simulink model "partH"  (R2018b)
settings: Solver=VariableStepAuto  StartTime=0.0  StopTime=10.0  RelTol=1e-3
settings Model: Creator=amir  LastModifiedBy=amir

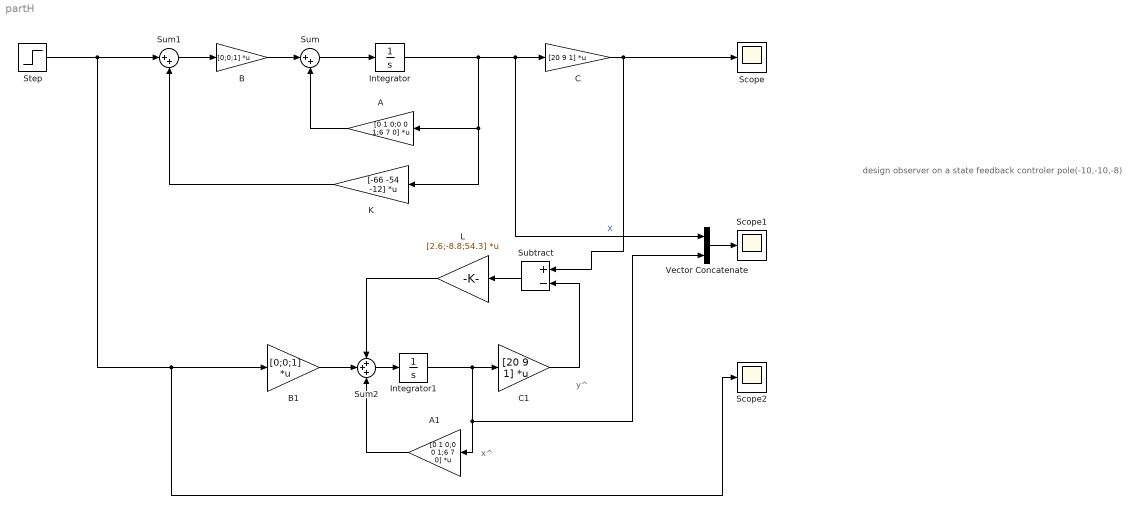
== system partH ==
  note: design observer on a
      | state feedback controler
      | pole(-10,-10,-8)
  note: x^
  note: y^
  A : Gain  Gain=[0 1 0;0 0 1;6 7 0]  Multiplication=Matrix(K*u) (u vector)
  A1 : Gain  Gain=[0 1 0;0 0 1;6 7 0]  Multiplication=Matrix(K*u) (u vector)
  B : Gain  Gain=[0;0;1]  Multiplication=Matrix(K*u) (u vector)
  B1 : Gain  Gain=[0;0;1]  Multiplication=Matrix(K*u) (u vector)
  C : Gain  Gain=[20 9 1]  Multiplication=Matrix(K*u) (u vector)
  C1 : Gain  Gain=[20 9 1]  Multiplication=Matrix(K*u) (u vector)
  Integrator : Integrator  InitialCondition=[1;1;1]
  Integrator1 : Integrator  InitialCondition=[1;1;1]
  K : Gain  Gain=[-66 -54 -12]  Multiplication=Matrix(K*u) (u vector)
  L : Gain  Gain=[2.6;-8.8;54.3]  Multiplication=Matrix(K*u) (u vector)
  Scope : Scope
  Scope1 : Scope
  Scope2 : Scope
  Step : Step  SampleTime=0
  Subtract : Sum  Inputs=+-
  Sum : Sum  Inputs=|++
  Sum1 : Sum  Inputs=|++
  Sum2 : Sum  Inputs=+++
  Vector Concatenate : Concatenate
  wires:
  Step/1 -> Scope2/1, B1/1, Sum1/1
  K/1 -> Sum1/2
  Sum1/1 -> B/1
  Integrator/1 -> Vector Concatenate/1, C/1, K/1, A/1  "X"
  Sum/1 -> Integrator/1
  C/1 -> Scope/1, Subtract/1
  A/1 -> Sum/2
  B/1 -> Sum/1
  B1/1 -> Sum2/2
  Sum2/1 -> Integrator1/1
  Vector Concatenate/1 -> Scope1/1
  A1/1 -> Sum2/3
  Integrator1/1 -> C1/1, Vector Concatenate/2, A1/1
  C1/1 -> Subtract/2
  Subtract/1 -> L/1
  L/1 -> Sum2/1
